simulink model "es7"  (R2022b)
settings: Solver=VariableStepAuto  StartTime=0.0  StopTime=10.0  RelTol=1e-3
settings Model: Creator=adlercohen  LastModifiedBy=adlercohen

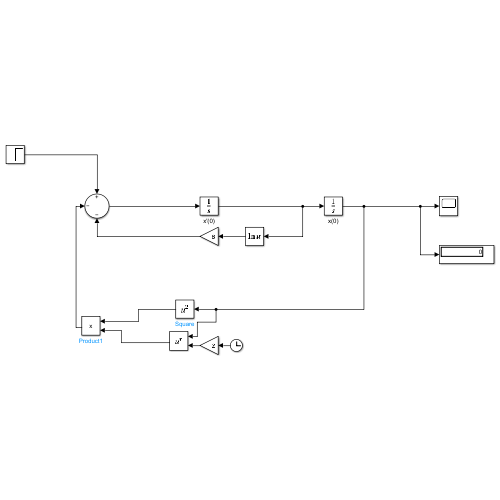
[thumbnail: Simulink's stored preview of the top-level diagram]
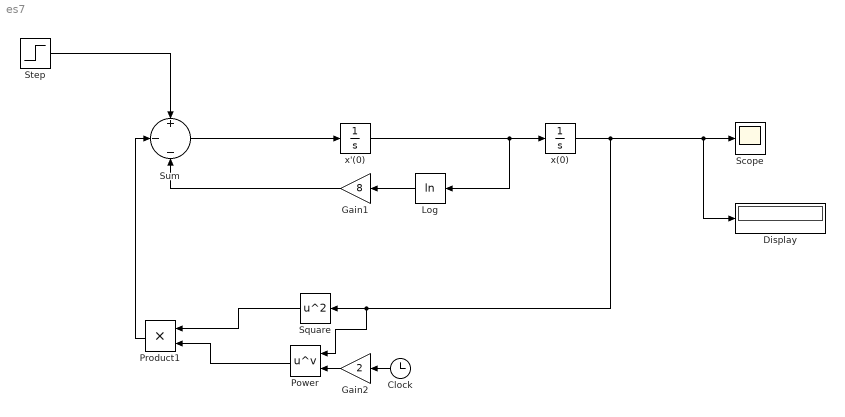
== system es7 ==
  Clock : Clock
  Display : Display
  Gain1 : Gain  Gain=8
  Gain2 : Gain  Gain=2
  Log : Math  Operator=log
  Power : Math  Operator=pow
  Product1 : Product
  Scope : Scope
  Square : Math  Operator=square
  Step : Step  Time=0  SampleTime=0
  Sum : Sum  Inputs=+|-|-
  x'(0) : Integrator
  x(0) : Integrator
  wires:
  Clock/1 -> Gain2/1
  x'(0)/1 -> Log/1, x(0)/1
  x(0)/1 -> Power/1, Square/1, Scope/1, Display/1
  Gain1/1 -> Sum/3
  Step/1 -> Sum/1
  Sum/1 -> x'(0)/1
  Log/1 -> Gain1/1
  Square/1 -> Product1/1
  Gain2/1 -> Power/2
  Power/1 -> Product1/2
  Product1/1 -> Sum/2
